simulink model "SPath"  (R2020a)
settings: Solver=VariableStepAuto  StartTime=0.0  StopTime=150  RelTol=1e-3
values from neighbouring files (symbols this model uses):
  b = 0.4    [Takeoff.m]
  body_rate_0 = [0;0;0]    [Takeoff.m]
  Boundaries = [B1;B2;B3]    [Takeoff.m]
  Euler_0 = [0;0;0]    [Takeoff.m]
  g = [0;0;-9.8]    [Takeoff.m]
  I_Drone = [0.3933,0.3933,0.76]    [Takeoff.m]
  I_Tank = CalItank(m_tank,0.4,0.1,0.4,i)    [Takeoff.m]
  J = 0.00062    [Takeoff.m]
  K = 0.074    [Takeoff.m]
  k_T = MaxMotorThrsut/(MaxRPM^2)    (= 6.99167657551e-06)    [Takeoff.m]
  k_Thrsut2Torque = 0.021    [Takeoff.m]
  l = 0.5    [Takeoff.m]
  L = sqrt((x2-x1)^2 + (y2-y1)^2)    [Takeoff.m]
  m = m_drone + m_tank*percent    (= 36)    [Takeoff.m]    (also in animation.m = T_V1toI*T_V2toV1*T_BtoV2)
  m_drone = 20    [Takeoff.m]
  m_tank = 16    [Takeoff.m]
  MaxThrust = 4*MaxMotorThrsut    (= 529.2)    [Takeoff.m]
  MaxTilt = 30*pi/180    (= 0.523598775598)    [Takeoff.m]
  MaxTorque_XY = (T2-T1)*(l/sqrt(2))    [Takeoff.m]
  MaxVolt = 48    [Takeoff.m]
  MaxYawRate = 100*pi/180    (= 1.74532925199)    [Takeoff.m]
  MaxZVel = 2    [Takeoff.m]
  percent = 1    [Takeoff.m]
  Px1 = 0.2    [Takeoff.m]
  Pz1 = 1    [Takeoff.m]
  Pz2 = 100    [Takeoff.m]
  R = 0.0062    [Takeoff.m]
  SafeZone = 1.0    (= 1)    [Takeoff.m]
  ts = 0.01    [Takeoff.m]
  WayPts = [[XYZ_0(1) XYZ_0(2) XYZ_0(3)] ... (first row only)    [Takeoff.m]
  XYZ_0 = [0;0;0]    [Takeoff.m]
undefined symbols (not defined in the file or in its folder): b_tank, d_drone, d_tank, DiscIntNeverNeededParam, FlyVel, h_tank, NWay, PD1, PD2, PI1, PI2, PP1, PP2, Sensor0Dir, ts_out, WayPtsYaw
libraries: simulink x26, vrlib x4, simulink_extras x2
(part 3 of 3)

== system SPath/Controller/Rotors System1/Propellers/Motor Thrust Control2 ==
  Ref_Thrust : Inport
  DC Motor : Subsystem
  Gain2 : Gain  Gain=k_T
  Gain3 : Gain  Gain=1/k_T
  Gain4 : Gain  Gain=30/pi
  MATLAB Function : MATLAB Function  TreatAsAtomicUnit=on
  PID Controller : simulink/Continuous/PID Controller  Controller=PI  Form=Parallel  TimeDomain=Discrete-time  UseExternalTs=off  SampleTime=ts  IntegratorMethod=Forward Euler  FilterMethod=Forward Euler  ControllerParametersSource=internal  P=0.005  I=0.5  D=0.01  UseFilter=on  N=100  TunerSelectOption=Transfer Function Based (PID Tuner App)  InitialConditionSource=internal  InitialConditionForIntegrator=0  InitialConditionForFilter=0  DifferentiatorICPrevScaledInput=0  ExternalReset=none  TrackingMode=off  Kt=1  LimitOutput=off  UpperSaturationLimit=inf  LowerSaturationLimit=-inf  LinearizeAsGain=on  AntiWindupMode=none  Kb=1  POutMin=[]  POutMax=[]  IOutMin=[]  IOutMax=[]  DOutMin=[]  DOutMax=[]  NOutMin=[]  NOutMax=[]  SumOutMin=[]  SumOutMax=[]  SaturationOutMin=[]  SaturationOutMax=[]  PParamMin=[]  PParamMax=[]  IParamMin=[]  IParamMax=[]  DParamMin=[]  DParamMax=[]  NParamMin=[]  NParamMax=[]  KbParamMin=[]  KbParamMax=[]  KtParamMin=[]  KtParamMax=[]  KbOutMin=[]  KbOutMax=[]  KtOutMin=[]  KtOutMax=[]  IntegratorOutMin=[]  IntegratorOutMax=[]  FilterOutMin=[]  FilterOutMax=[]  SumI1OutMin=[]  SumI1OutMax=[]  SumI2OutMin=[]  SumI2OutMax=[]  SumI3OutMin=[]  SumI3OutMax=[]  SumI4OutMin=[]  SumI4OutMax=[]  SumDOutMin=[]  SumDOutMax=[]  DifferentiatorOutMin=[]  DifferentiatorOutMax=[]  FilterDiffOutCoefMin=[]  FilterDiffOutCoefMax=[]  ReciprocalOutMin=[]  ReciprocalOutMax=[]  SumDenOutMin=[]  SumDenOutMax=[]  SumNumOutMin=[]  SumNumOutMax=[]  DivideOutMin=[]  DivideOutMax=[]  UdiffTsProdOutMin=[]  UdiffTsProdOutMax=[]  NTsProdOutMin=[]  NTsProdOutMax=[]  UintegralTsProdOutMin=[]  UintegralTsProdOutMax=[]  UngainTsProdOutMin=[]  UngainTsProdOutMax=[]  IntegratorContinuousStateAttributes=''  IntegratorStateMustResolveToSignalObject=off  IntegratorRTWStateStorageClass=Auto  FilterContinuousStateAttributes=''  FilterStateMustResolveToSignalObject=off  FilterRTWStateStorageClass=Auto  ParallelPVariant=InternalParameters  IdealPVariant=Disabled  IVariant=InternalParameters  DVariant=Disabled  IntegratorVariant=Discrete  SatVariant=Disabled  AWVariant=Passthrough  PCopyVariant=Disabled  TRVariant=Disabled  FdbkBlocksVariant=Forward  IdealPFdbkVariant=Disabled  SatFdbkVariant=Disabled  DerivativeFilterVariant=Disabled  NVariant=Disabled  NCopyVariant=Disabled_SignalSpec  FilterICVariant=Disabled  IntegratorICVariant=InternalICs  ExternalResetVariant=Disabled  TRSumVariant=Passthrough  SumFdbkVariant=Disabled  SumVariant=Sum_PI  TsampFilterVariant=InternalTs  TsampNgainVariant=Passthrough  TsampIntegralVariant=Passthrough
  PID Controller1 : simulink/Continuous/PID Controller  Commented=on  Controller=PID  Form=Parallel  TimeDomain=Discrete-time  UseExternalTs=off  SampleTime=ts  IntegratorMethod=Forward Euler  FilterMethod=Forward Euler  ControllerParametersSource=internal  P=69.4635476284255  I=231.449566152495  D=-0.149403920537339  UseFilter=on  N=139.13500041138  TunerSelectOption=Transfer Function Based (PID Tuner App)  InitialConditionSource=internal  InitialConditionForIntegrator=0  InitialConditionForFilter=0  DifferentiatorICPrevScaledInput=0  ExternalReset=none  TrackingMode=off  Kt=1  LimitOutput=off  UpperSaturationLimit=inf  LowerSaturationLimit=-inf  LinearizeAsGain=on  AntiWindupMode=none  Kb=1  POutMin=[]  POutMax=[]  IOutMin=[]  IOutMax=[]  DOutMin=[]  DOutMax=[]  NOutMin=[]  NOutMax=[]  SumOutMin=[]  SumOutMax=[]  SaturationOutMin=[]  SaturationOutMax=[]  PParamMin=[]  PParamMax=[]  IParamMin=[]  IParamMax=[]  DParamMin=[]  DParamMax=[]  NParamMin=[]  NParamMax=[]  KbParamMin=[]  KbParamMax=[]  KtParamMin=[]  KtParamMax=[]  KbOutMin=[]  KbOutMax=[]  KtOutMin=[]  KtOutMax=[]  IntegratorOutMin=[]  IntegratorOutMax=[]  FilterOutMin=[]  FilterOutMax=[]  SumI1OutMin=[]  SumI1OutMax=[]  SumI2OutMin=[]  SumI2OutMax=[]  SumI3OutMin=[]  SumI3OutMax=[]  SumI4OutMin=[]  SumI4OutMax=[]  SumDOutMin=[]  SumDOutMax=[]  DifferentiatorOutMin=[]  DifferentiatorOutMax=[]  FilterDiffOutCoefMin=[]  FilterDiffOutCoefMax=[]  ReciprocalOutMin=[]  ReciprocalOutMax=[]  SumDenOutMin=[]  SumDenOutMax=[]  SumNumOutMin=[]  SumNumOutMax=[]  DivideOutMin=[]  DivideOutMax=[]  UdiffTsProdOutMin=[]  UdiffTsProdOutMax=[]  NTsProdOutMin=[]  NTsProdOutMax=[]  UintegralTsProdOutMin=[]  UintegralTsProdOutMax=[]  UngainTsProdOutMin=[]  UngainTsProdOutMax=[]  IntegratorContinuousStateAttributes=''  IntegratorStateMustResolveToSignalObject=off  IntegratorRTWStateStorageClass=Auto  FilterContinuousStateAttributes=''  FilterStateMustResolveToSignalObject=off  FilterRTWStateStorageClass=Auto  ParallelPVariant=InternalParameters  IdealPVariant=Disabled  IVariant=InternalParameters  DVariant=InternalParameters  IntegratorVariant=Discrete  SatVariant=Disabled  AWVariant=Passthrough  PCopyVariant=Disabled  TRVariant=Disabled  FdbkBlocksVariant=Forward  IdealPFdbkVariant=Disabled  SatFdbkVariant=Disabled  DerivativeFilterVariant=ForwardEulerFilter  NVariant=InternalParameters  NCopyVariant=Disabled  FilterICVariant=InternalICsFilter  IntegratorICVariant=InternalICs  ExternalResetVariant=Disabled  TRSumVariant=Passthrough  SumFdbkVariant=Disabled  SumVariant=Sum_PID  TsampFilterVariant=InternalTs  TsampNgainVariant=Passthrough  TsampIntegralVariant=Passthrough
  Rate Transition : RateTransition  OutPortSampleTime=ts
  Saturation1 : Saturate  Commented=on  UpperLimit=MaxVolt  LowerLimit=-MaxVolt
  Scope : Scope
  Scope1 : Scope
  Square : Math  Operator=square  SaturateOnIntegerOverflow=on
  Square Root : Sqrt  SaturateOnIntegerOverflow=on
  Sum : Sum  Inputs=|+-
  Transfer Fcn1 : TransferFcn  Commented=on  Numerator=[44 44]  Denominator=[1 0.01]
  Thrust : Outport
  wires:
  MATLAB Function/1(y) -> DC Motor/2(TQ_load)
  Sum/1 -> PID Controller/1
  Square Root/1 -> Sum/1  "Ref_RPM"
  PID Controller/1 -> DC Motor/1(Voltage)
  Gain4/1 -> Scope/1, Square/1, Rate Transition/1, MATLAB Function/1(u)  "RPM"
  DC Motor/1(Speed) -> Gain4/1
  Rate Transition/1 -> Sum/2
  Gain2/1 -> Thrust/1, Scope1/1  "Thrust"
  Ref_Thrust/1 -> Gain3/1
  Square/1 -> Gain2/1
  Gain3/1 -> Square Root/1

== system SPath/Controller/Rotors System1/Propellers/Motor Thrust Control3 ==
  Ref_Thrust : Inport
  DC Motor : Subsystem
  Gain2 : Gain  Gain=k_T
  Gain3 : Gain  Gain=1/k_T
  Gain4 : Gain  Gain=30/pi
  MATLAB Function : MATLAB Function  TreatAsAtomicUnit=on
  PID Controller : simulink/Continuous/PID Controller  Controller=PI  Form=Parallel  TimeDomain=Discrete-time  UseExternalTs=off  SampleTime=ts  IntegratorMethod=Forward Euler  FilterMethod=Forward Euler  ControllerParametersSource=internal  P=0.005  I=0.5  D=0.01  UseFilter=on  N=100  TunerSelectOption=Transfer Function Based (PID Tuner App)  InitialConditionSource=internal  InitialConditionForIntegrator=0  InitialConditionForFilter=0  DifferentiatorICPrevScaledInput=0  ExternalReset=none  TrackingMode=off  Kt=1  LimitOutput=off  UpperSaturationLimit=inf  LowerSaturationLimit=-inf  LinearizeAsGain=on  AntiWindupMode=none  Kb=1  POutMin=[]  POutMax=[]  IOutMin=[]  IOutMax=[]  DOutMin=[]  DOutMax=[]  NOutMin=[]  NOutMax=[]  SumOutMin=[]  SumOutMax=[]  SaturationOutMin=[]  SaturationOutMax=[]  PParamMin=[]  PParamMax=[]  IParamMin=[]  IParamMax=[]  DParamMin=[]  DParamMax=[]  NParamMin=[]  NParamMax=[]  KbParamMin=[]  KbParamMax=[]  KtParamMin=[]  KtParamMax=[]  KbOutMin=[]  KbOutMax=[]  KtOutMin=[]  KtOutMax=[]  IntegratorOutMin=[]  IntegratorOutMax=[]  FilterOutMin=[]  FilterOutMax=[]  SumI1OutMin=[]  SumI1OutMax=[]  SumI2OutMin=[]  SumI2OutMax=[]  SumI3OutMin=[]  SumI3OutMax=[]  SumI4OutMin=[]  SumI4OutMax=[]  SumDOutMin=[]  SumDOutMax=[]  DifferentiatorOutMin=[]  DifferentiatorOutMax=[]  FilterDiffOutCoefMin=[]  FilterDiffOutCoefMax=[]  ReciprocalOutMin=[]  ReciprocalOutMax=[]  SumDenOutMin=[]  SumDenOutMax=[]  SumNumOutMin=[]  SumNumOutMax=[]  DivideOutMin=[]  DivideOutMax=[]  UdiffTsProdOutMin=[]  UdiffTsProdOutMax=[]  NTsProdOutMin=[]  NTsProdOutMax=[]  UintegralTsProdOutMin=[]  UintegralTsProdOutMax=[]  UngainTsProdOutMin=[]  UngainTsProdOutMax=[]  IntegratorContinuousStateAttributes=''  IntegratorStateMustResolveToSignalObject=off  IntegratorRTWStateStorageClass=Auto  FilterContinuousStateAttributes=''  FilterStateMustResolveToSignalObject=off  FilterRTWStateStorageClass=Auto  ParallelPVariant=InternalParameters  IdealPVariant=Disabled  IVariant=InternalParameters  DVariant=Disabled  IntegratorVariant=Discrete  SatVariant=Disabled  AWVariant=Passthrough  PCopyVariant=Disabled  TRVariant=Disabled  FdbkBlocksVariant=Forward  IdealPFdbkVariant=Disabled  SatFdbkVariant=Disabled  DerivativeFilterVariant=Disabled  NVariant=Disabled  NCopyVariant=Disabled_SignalSpec  FilterICVariant=Disabled  IntegratorICVariant=InternalICs  ExternalResetVariant=Disabled  TRSumVariant=Passthrough  SumFdbkVariant=Disabled  SumVariant=Sum_PI  TsampFilterVariant=InternalTs  TsampNgainVariant=Passthrough  TsampIntegralVariant=Passthrough
  PID Controller1 : simulink/Continuous/PID Controller  Commented=on  Controller=PID  Form=Parallel  TimeDomain=Discrete-time  UseExternalTs=off  SampleTime=ts  IntegratorMethod=Forward Euler  FilterMethod=Forward Euler  ControllerParametersSource=internal  P=69.4635476284255  I=231.449566152495  D=-0.149403920537339  UseFilter=on  N=139.13500041138  TunerSelectOption=Transfer Function Based (PID Tuner App)  InitialConditionSource=internal  InitialConditionForIntegrator=0  InitialConditionForFilter=0  DifferentiatorICPrevScaledInput=0  ExternalReset=none  TrackingMode=off  Kt=1  LimitOutput=off  UpperSaturationLimit=inf  LowerSaturationLimit=-inf  LinearizeAsGain=on  AntiWindupMode=none  Kb=1  POutMin=[]  POutMax=[]  IOutMin=[]  IOutMax=[]  DOutMin=[]  DOutMax=[]  NOutMin=[]  NOutMax=[]  SumOutMin=[]  SumOutMax=[]  SaturationOutMin=[]  SaturationOutMax=[]  PParamMin=[]  PParamMax=[]  IParamMin=[]  IParamMax=[]  DParamMin=[]  DParamMax=[]  NParamMin=[]  NParamMax=[]  KbParamMin=[]  KbParamMax=[]  KtParamMin=[]  KtParamMax=[]  KbOutMin=[]  KbOutMax=[]  KtOutMin=[]  KtOutMax=[]  IntegratorOutMin=[]  IntegratorOutMax=[]  FilterOutMin=[]  FilterOutMax=[]  SumI1OutMin=[]  SumI1OutMax=[]  SumI2OutMin=[]  SumI2OutMax=[]  SumI3OutMin=[]  SumI3OutMax=[]  SumI4OutMin=[]  SumI4OutMax=[]  SumDOutMin=[]  SumDOutMax=[]  DifferentiatorOutMin=[]  DifferentiatorOutMax=[]  FilterDiffOutCoefMin=[]  FilterDiffOutCoefMax=[]  ReciprocalOutMin=[]  ReciprocalOutMax=[]  SumDenOutMin=[]  SumDenOutMax=[]  SumNumOutMin=[]  SumNumOutMax=[]  DivideOutMin=[]  DivideOutMax=[]  UdiffTsProdOutMin=[]  UdiffTsProdOutMax=[]  NTsProdOutMin=[]  NTsProdOutMax=[]  UintegralTsProdOutMin=[]  UintegralTsProdOutMax=[]  UngainTsProdOutMin=[]  UngainTsProdOutMax=[]  IntegratorContinuousStateAttributes=''  IntegratorStateMustResolveToSignalObject=off  IntegratorRTWStateStorageClass=Auto  FilterContinuousStateAttributes=''  FilterStateMustResolveToSignalObject=off  FilterRTWStateStorageClass=Auto  ParallelPVariant=InternalParameters  IdealPVariant=Disabled  IVariant=InternalParameters  DVariant=InternalParameters  IntegratorVariant=Discrete  SatVariant=Disabled  AWVariant=Passthrough  PCopyVariant=Disabled  TRVariant=Disabled  FdbkBlocksVariant=Forward  IdealPFdbkVariant=Disabled  SatFdbkVariant=Disabled  DerivativeFilterVariant=ForwardEulerFilter  NVariant=InternalParameters  NCopyVariant=Disabled  FilterICVariant=InternalICsFilter  IntegratorICVariant=InternalICs  ExternalResetVariant=Disabled  TRSumVariant=Passthrough  SumFdbkVariant=Disabled  SumVariant=Sum_PID  TsampFilterVariant=InternalTs  TsampNgainVariant=Passthrough  TsampIntegralVariant=Passthrough
  Rate Transition : RateTransition  OutPortSampleTime=ts
  Saturation1 : Saturate  Commented=on  UpperLimit=MaxVolt  LowerLimit=-MaxVolt
  Scope : Scope
  Scope1 : Scope
  Square : Math  Operator=square  SaturateOnIntegerOverflow=on
  Square Root : Sqrt  SaturateOnIntegerOverflow=on
  Sum : Sum  Inputs=|+-
  Transfer Fcn1 : TransferFcn  Commented=on  Numerator=[44 44]  Denominator=[1 0.01]
  Thrust : Outport
  wires:
  Gain3/1 -> Square Root/1
  Square/1 -> Gain2/1
  Ref_Thrust/1 -> Gain3/1
  Gain2/1 -> Scope1/1, Thrust/1  "Thrust"
  Rate Transition/1 -> Sum/2
  DC Motor/1(Speed) -> Gain4/1
  Gain4/1 -> MATLAB Function/1(u), Rate Transition/1, Square/1, Scope/1  "RPM"
  PID Controller/1 -> DC Motor/1(Voltage)
  Square Root/1 -> Sum/1  "Ref_RPM"
  Sum/1 -> PID Controller/1
  MATLAB Function/1(y) -> DC Motor/2(TQ_load)

== system SPath/Controller/Rotors System1/Propellers/Motor Thrust Control/Brushless DC Motor ==
  note: d2/dt2(theta)
  note: d/dt(theta)
  note: d/dt(i)
  note: i
  Voltage : Inport
  TQ_load : Inport  Port=2
  Add : Sum  Inputs=-+-
  Add1 : Sum  Inputs=+--
  Damping : Gain  Gain=b
  Inductance : Gain  Gain=1/L
  Inertia : Gain  Gain=1/J
  Integrator : Integrator
  Integrator1 : Integrator
  Ke : Gain  Gain=K
  Kt : Gain  Gain=K
  Resistance : Gain  Gain=R
  Scope : Scope  NumInputPorts=2
  Speed : Outport
  wires:
  TQ_load/1 -> Add1/3
  Add1/1 -> Inertia/1
  Add/1 -> Inductance/1
  Ke/1 -> Add/3
  Damping/1 -> Add1/2
  Resistance/1 -> Add/1
  Voltage/1 -> Add/2
  Kt/1 -> Add1/1
  Integrator/1 -> Resistance/1, Scope/1, Kt/1
  Inertia/1 -> Integrator1/1
  Integrator1/1 -> Ke/1, Speed/1, Scope/2, Damping/1
  Inductance/1 -> Integrator/1

== system SPath/Controller/Rotors System1/Propellers/Motor Thrust Control1/DC Motor ==
  note: i
  note: d/dt(i)
  note: d/dt(theta)
  note: d2/dt2(theta)
  Voltage : Inport
  TQ_load : Inport  Port=2
  Add : Sum  Inputs=-+-
  Add1 : Sum  Inputs=+--
  Damping : Gain  Gain=b
  Inductance : Gain  Gain=1/L
  Inertia : Gain  Gain=1/J
  Integrator : Integrator
  Integrator1 : Integrator
  Ke : Gain  Gain=K
  Kt : Gain  Gain=K
  Resistance : Gain  Gain=R
  Scope : Scope  NumInputPorts=2
  Speed : Outport
  wires:
  Inductance/1 -> Integrator/1
  Integrator1/1 -> Damping/1, Scope/2, Speed/1, Ke/1
  Inertia/1 -> Integrator1/1
  Integrator/1 -> Kt/1, Scope/1, Resistance/1
  Kt/1 -> Add1/1
  Voltage/1 -> Add/2
  Resistance/1 -> Add/1
  Damping/1 -> Add1/2
  Ke/1 -> Add/3
  Add/1 -> Inductance/1
  Add1/1 -> Inertia/1
  TQ_load/1 -> Add1/3

== system SPath/Controller/Rotors System1/Propellers/Motor Thrust Control2/DC Motor ==
  note: d2/dt2(theta)
  note: d/dt(theta)
  note: d/dt(i)
  note: i
  Voltage : Inport
  TQ_load : Inport  Port=2
  Add : Sum  Inputs=-+-
  Add1 : Sum  Inputs=+--
  Damping : Gain  Gain=b
  Inductance : Gain  Gain=1/L
  Inertia : Gain  Gain=1/J
  Integrator : Integrator
  Integrator1 : Integrator
  Ke : Gain  Gain=K
  Kt : Gain  Gain=K
  Resistance : Gain  Gain=R
  Scope : Scope  NumInputPorts=2
  Speed : Outport
  wires:
  TQ_load/1 -> Add1/3
  Add1/1 -> Inertia/1
  Add/1 -> Inductance/1
  Ke/1 -> Add/3
  Damping/1 -> Add1/2
  Resistance/1 -> Add/1
  Voltage/1 -> Add/2
  Kt/1 -> Add1/1
  Integrator/1 -> Resistance/1, Scope/1, Kt/1
  Inertia/1 -> Integrator1/1
  Integrator1/1 -> Ke/1, Speed/1, Scope/2, Damping/1
  Inductance/1 -> Integrator/1

== system SPath/Controller/Rotors System1/Propellers/Motor Thrust Control3/DC Motor ==
  note: i
  note: d/dt(i)
  note: d/dt(theta)
  note: d2/dt2(theta)
  Voltage : Inport
  TQ_load : Inport  Port=2
  Add : Sum  Inputs=-+-
  Add1 : Sum  Inputs=+--
  Damping : Gain  Gain=b
  Inductance : Gain  Gain=1/L
  Inertia : Gain  Gain=1/J
  Integrator : Integrator
  Integrator1 : Integrator
  Ke : Gain  Gain=K
  Kt : Gain  Gain=K
  Resistance : Gain  Gain=R
  Scope : Scope  NumInputPorts=2
  Speed : Outport
  wires:
  Inductance/1 -> Integrator/1
  Integrator1/1 -> Damping/1, Scope/2, Speed/1, Ke/1
  Inertia/1 -> Integrator1/1
  Integrator/1 -> Kt/1, Scope/1, Resistance/1
  Kt/1 -> Add1/1
  Voltage/1 -> Add/2
  Resistance/1 -> Add/1
  Damping/1 -> Add1/2
  Ke/1 -> Add/3
  Add/1 -> Inductance/1
  Add1/1 -> Inertia/1
  TQ_load/1 -> Add1/3

== matlab function SPath/Controller/Rotors System1/Propellers/Motor Thrust Control/MATLAB Function ==
  data: u input; y output
function y = fcn(u)
    y = 0.000009*u^2;

    % The coefficient is decided by experimental value.
    % Max RPM = 4350, 48 Volt.

== matlab function SPath/Controller/Rotors System1/Propellers/Motor Thrust Control1/MATLAB Function ==
  data: u input; y output
function y = fcn(u)
    y = 0.000009*u^2;

    % The coefficient is decided by experimental value.
    % Max RPM = 4350, 48 Volt.

== matlab function SPath/Controller/Rotors System1/Propellers/Motor Thrust Control2/MATLAB Function ==
  data: u input; y output
function y = fcn(u)
    y = 0.000009*u^2;

    % The coefficient is decided by experimental value.
    % Max RPM = 4350, 48 Volt.

== matlab function SPath/6dof_system/Drone & Liquid Dynamic Inertia/DroneTankI ==
  data: I_D input; I output; I_T input; M_D input; M_T input; Z_D input; Z_T input; CR_X input; CR_Y input
function I = fcn(I_D,I_T,M_D,M_T,Z_D,Z_T,CR_X,CR_Y)

    Ix = I_D(1) + M_D*Z_D^2 + CR_X*I_T(1) + M_T*Z_T^2;
    Iy = I_D(2) + M_D*Z_D^2 + CR_Y*I_T(2) + M_T*Z_T^2;
    Iz = I_D(3) + I_T(3);
    I = [[Ix 0 0];[0 Iy 0];[0 0 Iz]];

== matlab function SPath/6dof_system/Drone & Liquid Dynamic Inertia/FullTankCR ==
  data: w_d input; CR_x output; CR_y output; C_R input
function [CR_x,CR_y] = fcn(w_d,C_R)
if length(w_d) > 1
    if abs(w_d(2)) > 0.001
        CR_y = C_R;
    else
        CR_y = 1;
    end
    
    if abs(w_d(1)) > 0.001
        CR_x = C_R;
    else
        CR_x = 1;
    end
else
    CR_x = 1;
    CR_y = 1;
end

== matlab function SPath/Controller/Rotors System1/Propellers/Motor Thrust Control3/MATLAB Function ==
  data: u input; y output
function y = fcn(u)
    y = 0.000009*u^2;

    % The coefficient is decided by experimental value.
    % Max RPM = 4350, 48 Volt.

== matlab function SPath/Controller/ActionDecider/SlowDown_Detect/SlowDown_Detect ==
  data: mode input; D_SD input; D_SF input; S0X input; action output; S0Y input; S1X input; S2X input
function action = fcn(mode,D_SD,D_SF,S0X,S0Y,S1X,S2X)
action = 0;
if mode == 0     
    
    if abs(S0X) <= D_SD && abs(S0Y) <= 1.5*D_SF
        action = 1;
    end
    
end

== matlab function SPath/Controller/Sensors/Sensor0 (15 degree sensor) ==
  data: Pos input; MinBDist output; Bounds input; Yaw input; MinBVect output; Directions input; RightVect output; MinRight output; LeftVect output; MinLeft output
function [MinBDist,MinBVect,RightVect,MinRight,LeftVect,MinLeft] = fcn(Pos,Bounds,Yaw,Directions)
MaxRange = 30;
MinBDist = MaxRange;
m = [[cos(Yaw) -sin(Yaw)];[sin(Yaw) cos(Yaw)]];
nn = m*[1;0];
MinBVect = [nn(1);nn(2);0];

% For Visual
RightVect = MinBVect;
MinRight = MaxRange;
LeftVect = MinBVect;
MinLeft = MaxRange;

RightDist = MaxRange;
LeftDist = MaxRange;

for b = 1:size(Bounds,1)
Bound = Bounds(b,:);

%Bound = Bounds(BIndex,:);
MinSenseDist = MaxRange;
m = [[cos(Yaw) -sin(Yaw)];[sin(Yaw) cos(Yaw)]];
nnn = m*[1;0];
MinSenseVect = [nnn(1);nnn(2);0];




for k = 1:size(Directions,2)
if length(Pos) > 1
    bx = Bound(1);
    by = Bound(2);
    tx = Bound(3);
    ty = Bound(4);
    X = Pos(1);
    Y = Pos(2);
    Z = Pos(3);
    
    m = [[cos(Yaw) -sin(Yaw)];[sin(Yaw) cos(Yaw)]];
    nn = m*Directions(:,k); % Sense vector in Inertia Frame
    nx = nn(1);
    ny = nn(2);

    j = ((ty*bx-tx*by)-(ty*X-tx*Y))/(ty*nx-tx*ny);
    
    if j < 0 % sense backward point
        SenseDist = MaxRange;
    else
        SensePt = [X+nx*j;Y+ny*j];
        
        % Check if ON boundaries
        if tx == 0
            i = (SensePt(2)-by)/ty;
        else
            i = (SensePt(1)-bx)/tx;
        end
        
        % If not
        if i < 0 || i > Bound(7)
            SenseDist = MaxRange;
        % If yes
        else
            SenseDist = sqrt((nx*j)^2 + (ny*j)^2);
        end
    end
    
    % Calculate Directions
    SenseVect = [nx;ny;0]/sqrt(nx^2+ny^2);
    
else
    SenseDist = MaxRange;
    SenseVect = [0;0;0];
end

if SenseDist < MinSenseDist
    MinSenseDist = SenseDist;
    MinSenseVect = SenseVect;
end

% Collect Right and Left Bounds Vector for Visual
if k == 1
    RightVect = SenseVect;
    RightDist = SenseDist;
end
if k == size(Directions,2)
    LeftVect = SenseVect;
    LeftDist = SenseDist;
end


end % end of -15:1:15 for loop


if MinSenseDist < MinBDist
    MinBDist = MinSenseDist;
    MinBVect = MinSenseVect;
end


if RightDist < MinRight
    MinRight = RightDist;
end

if LeftDist < MinLeft
    MinLeft = LeftDist;
end


end

== matlab function SPath/Controller/FlyModeCmd/SlowDown Fly ==
  data: mode input; XVelCmd output; V_AO input
function XVelCmd = fcn(mode,V_AO)
% Mode 1: SlowDown Fly
XVelCmd = 0;
if mode == 1
    XVelCmd = V_AO;
end

== matlab function SPath/Controller/FlyModeCmd/FM Fly ==
  data: mode input; YVelCmd output; V_AO input; FM_Dir input
function YVelCmd = fcn(mode,V_AO,FM_Dir)
% Mode 2: First Maneuver Fly
YVelCmd = 0;
if mode == 2
    YVelCmd = FM_Dir*V_AO;
end

== matlab function SPath/Controller/Sensors/MATLAB Function ==
  data: Vect input; Vect_Body output; Yaw input
function Vect_Body = fcn(Vect,Yaw)
if length(Vect) > 1
    m = [[cos(Yaw) -sin(Yaw) 0];[sin(Yaw) cos(Yaw) 0]; [0 0 1]];
    m = transpose(m);
    Vect_Body = m*[Vect(1);Vect(2);0];
else
    Vect_Body = [1;0;0];
end

== matlab function SPath/Controller/ActionDecider/FirstManeuver_Detect/FM_Detect ==
  data: mode input; S0X input; S0Y input; action output; S1X input; S2X input; FM_Dir output; HotFix output; timeM1 input
function [action,FM_Dir,HotFix] = fcn(mode,S0X,S0Y,S1X,S2X,timeM1)
action = 0;
FM_Dir = 0;

MaxRange = 5;

%HotFix
HotFix = 0;

if mode == 1     
    if S0X <= 2.2 && timeM1 > 0.5 %2.5*D_SF + D_DR
        action = 1;
        
        % Decide Direction
        if S1X ~= MaxRange && S2X ~= MaxRange
            if S0Y < 0 % Something at Right
                FM_Dir = 1;    % Left Body Dir (1)
                HotFix = 1;
            else
                FM_Dir = -1;   % Right Body Dir
                HotFix = 1;
            end
            return;        
        end
        
        if S1X == MaxRange || S2X == MaxRange
            if S1X < MaxRange
                FM_Dir = 1; %(1 for left)
                HotFix = 1;
                
            elseif S2X < MaxRange
                FM_Dir = -1;
                HotFix = 1;
                
            else
                if S0Y < 0 % Something at Right
                    FM_Dir = 1;    % Left Body Dir (1)
                    
                    % Hot Fix for Extreme Case.
                    if abs(S0Y) >=  0.5*cos(45*pi/180)
                        HotFix = 1;
                    end
                else
                    FM_Dir = -1;   % Right Body Dir
                    
                    % Hot Fix for Extreme Case.
                    if abs(S0Y) >=  0.5*cos(45*pi/180)
                        HotFix = 1;
                    end
                end
            end
        end
        
    end  
    
    
    % Robust Algo: SlowDown but don't avoid: go to Normal Fly
    if S0X >= 20
        action = -1;
    end
    
end

== matlab function SPath/Controller/ActionDecider/SecondManeuver_Detect/XTouch_Detect ==
  data: mode input; Flag output; S1X input; S2X input; D_SF input; FM_Dir input
function Flag = fcn(mode,S1X,S2X,D_SF,FM_Dir)
Flag = 0;
if mode == 2
    if FM_Dir == -1 && S2X < 3*D_SF
        Flag = 1;
        return;
    end
    
    if FM_Dir == 1 && S1X < 3*D_SF
        Flag = 1;
        return;
    end
end

== matlab function SPath/6dof_system/BtoITransform ==
  data: phi input; m output; theta input; psi input
function m = fcn(phi,theta,psi)
    T_BtoV2 = [[1 0 0];[0 cos(-phi) sin(-phi)];[0 -sin(-phi) cos(-phi)]];
    T_V2toV1 = [[cos(-theta) 0 -sin(-theta)];[0 1 0];[sin(-theta) 0 cos(-theta)]];
    T_V1toI = [[cos(-psi) sin(-psi) 0];[-sin(-psi) cos(-psi) 0];[0 0 1]];
    m = T_V1toI*T_V2toV1*T_BtoV2;

== matlab function SPath/Controller/ActionDecider/SecondManeuver_Detect/SM_Detect ==
  data: mode input; timer1 input; action output; t_bf1 input
function action = fcn(mode,timer1,t_bf1)
action = 0;
if mode == 2 && timer1 >= t_bf1
    action = 1;
end

== matlab function SPath/Select WayPoint/ChooseTarget ==
  data: WayPts input; WayPtsYaw input; TargetWayPts output; WayPtsIndex input; TargetWayPtsYaw output; number input
function [TargetWayPts,TargetWayPtsYaw] = fcn(WayPts,WayPtsYaw,WayPtsIndex,number)
if WayPtsIndex < number
    TargetWayPts = WayPts(WayPtsIndex+1,:);
    TargetWayPtsYaw = WayPtsYaw(WayPtsIndex+1);
else
    TargetWayPts = WayPts(number,:);
    TargetWayPtsYaw = WayPtsYaw(number);
end

== matlab function SPath/Select WayPoint/IsReachTarget ==
  data: XYZe input; TouchWayPts output; Yawe input; Index input; time input; number input; Speed input
function TouchWayPts = fcn(XYZe,Yawe,Index,time,number,Speed)
TouchWayPts = 0;

if Index == 0
    if XYZe < 0.1
        TouchWayPts = 1;
    end
elseif Index == 1
    if time >= 5
        TouchWayPts = 1;
    end
elseif Index >= number
    TouchWayPts = 0;
else
    if XYZe < 0.1 && Yawe < 0.05 %&& Speed < 0.5
        TouchWayPts = 1;
    end  
end

== matlab function SPath/Controller/ActionDecider/SecondManeuver_Detect/Crossover_Detect ==
  data: mode input; IsTouchX input; S1X input; count output; S2X input; FM_Dir input; D_SF input
function count = fcn(mode,IsTouchX,S1X,S2X,FM_Dir,D_SF)
count = 0;

% HotFix
MaxRange = 5;

if mode == 2
if FM_Dir == -1
    if IsTouchX == 1 && S2X >= MaxRange
        count = 1;
        return;
    end
end

if FM_Dir == 1
    if IsTouchX == 1 && S1X >= MaxRange
        count = 1;
        return;
    end
end
end

== matlab function SPath/Controller/FlyModeCmd/SM Fly ==
  data: mode input; XVelCmd output; V_AO input
function XVelCmd = fcn(mode,V_AO)
% Mode 3: Second Maneuver Fly
XVelCmd = 0;
if mode == 3
    XVelCmd = V_AO;
end

== matlab function SPath/Controller/ActionDecider/Recover_Detect/Crossover_Detect ==
  data: mode input; IsTouchY input; S1Y input; count output; S2Y input; FM_Dir input; D_SF input
function count = fcn(mode,IsTouchY,S1Y,S2Y,FM_Dir,D_SF)
count = 0;
if mode == 3
if FM_Dir == -1
    if IsTouchY == 1 && S2Y > 2*D_SF
        count = 1;
        return;
    end
end

if FM_Dir == 1
    if IsTouchY == 1 && S1Y > 2*D_SF
        count = 1;
        return;
    end
end
end

== matlab function SPath/Controller/ActionDecider/Recover_Detect/TM_Detect ==
  data: mode input; timer2 input; action output; t_bf2 input
function action = fcn(mode,timer2,t_bf2)
action = 0;
if mode == 3 && timer2 >= t_bf2
    action = 1;
end

== matlab function SPath/Controller/ActionDecider/Recover_Detect/YTouch_Detect ==
  data: mode input; Flag output; S1Y input; S2Y input; D_SF input; FM_Dir input
function Flag = fcn(mode,S1Y,S2Y,D_SF,FM_Dir)
Flag = 0;
if mode == 3
    if FM_Dir == -1 && S2Y < 3*D_SF
        Flag = 1;
        return;
    end
    
    if FM_Dir == 1 && S1Y < 3*D_SF
        Flag = 1;
        return;
    end
end

== matlab function SPath/Controller/FlyModeCmd/Recover Fly ==
  data: mode input; YVelCmd output; V_AO input; FM_Dir input
function YVelCmd = fcn(mode,V_AO,FM_Dir)
% Mode 4: Recover Fly
YVelCmd = 0;
if mode == 4
    YVelCmd = -FM_Dir*V_AO;
end

== matlab function SPath/6dof_system/euler_rate ==
  data: p input; phi_d output; q input; r input; phi input; theta input; theta_d output; psi_d output; psi input
function [phi_d,theta_d,psi_d] = fcn(p,q,r,phi,theta,psi)
    D = [[1 sin(phi)*tan(theta) cos(phi)*tan(theta)];
         [0 cos(phi) -sin(phi)];
         [0 sin(phi)/cos(theta) cos(phi)/cos(theta)]];
    euler_rate = D*[p;q;r]
    phi_d = euler_rate(1)
    theta_d = euler_rate(2)
    psi_d = euler_rate(3)

== matlab function SPath/Controller/ActionDecider/IsRecoverFinish_Detect/MATLAB Function1 ==
  data: u input; y output
function y = fcn(u)
y = 0;
if u == 2
    y = 1;
end

== matlab function SPath/Controller/Sensors/MATLAB Function1 ==
  data: Pos_SensorX1 output; l input; Pos input; Pos_SensorX2 output; Pos_SensorY1 output; m_BtoI input; Pos_SensorY2 output
function [Pos_SensorX1,Pos_SensorX2,Pos_SensorY1,Pos_SensorY2] = fcn(l,Pos,m_BtoI)
    X = Pos(1);
    Y = Pos(2);
    Z = Pos(3);
    
    % Sensor X1 Place
    Sx1_B = [1;0;0]+[0;-1;0];
    Sx1_B = Sx1_B/norm(Sx1_B);
    Sx1_B = l*Sx1_B;
    
    Sx1_I = m_BtoI*Sx1_B;
    Pos_SensorX1 = [X+Sx1_I(1);Y+Sx1_I(2);Z+Sx1_I(3)];
    
    
    % Sensor X2 Place
    Sx2_B = [1;0;0]+[0;1;0];
    Sx2_B = Sx2_B/norm(Sx2_B);
    Sx2_B = l*Sx2_B;
    
    Sx2_I = m_BtoI*Sx2_B;
    Pos_SensorX2 = [X+Sx2_I(1);Y+Sx2_I(2);Z+Sx2_I(3)];
    
    % Sensor Y1 Place
    Sy1_B = [-1;0;0]+[0;-1;0];
    Sy1_B = Sy1_B/norm(Sy1_B);
    Sy1_B = l*Sy1_B;
    
    Sy1_I = m_BtoI*Sy1_B;
    Pos_SensorY1 = [X+Sy1_I(1);Y+Sy1_I(2);Z+Sy1_I(3)];
    
    
    % Sensor Y2 Place
    Sy2_B = [-1;0;0]+[0;1;0];
    Sy2_B = Sy2_B/norm(Sy2_B);
    Sy2_B = l*Sy2_B;
    
    Sy2_I = m_BtoI*Sy2_B;
    Pos_SensorY2 = [X+Sy2_I(1);Y+Sy2_I(2);Z+Sy2_I(3)];

== matlab function SPath/Controller/ActionDecider/IsRecoverFinish_Detect/MATLAB Function2 ==
  data: u input; y output
function y = fcn(u)
y = 0;
if u == 4
    y = 1;
end

== matlab function SPath/Controller/Sensors/SensorY2 ==
  data: Pos input; MinSenseDist output; Bounds input; Yaw input; SenseVect output; MaxRange input
function [MinSenseDist,SenseVect] = fcn(Pos,Bounds,Yaw,MaxRange)
MinSenseDist = MaxRange;
for index = 1:size(Bounds,1)
    Bound = Bounds(index,:);
if length(Pos) > 1
    bx = Bound(1);
    by = Bound(2);
    tx = Bound(3);
    ty = Bound(4);
    X = Pos(1);
    Y = Pos(2);
    Z = Pos(3);
    
    m = [[cos(Yaw) -sin(Yaw)];[sin(Yaw) cos(Yaw)]];
    n = m*[0;1]; % Yb vector
    nx = n(1);
    ny = n(2);

    j = ((ty*bx-tx*by)-(ty*X-tx*Y))/(ty*nx-tx*ny);
    
    if j < 0 % sense backward point
        SenseDist = MaxRange;
    else
        SensePt = [X+nx*j;Y+ny*j];
        
        % Check if ON boundaries
        if tx == 0
            i = (SensePt(2)-by)/ty;
        else
            i = (SensePt(1)-bx)/tx;
        end
        
        % If not
        if i < 0 || i > Bound(7)
            SenseDist = MaxRange;
        % If yes
        else
            SenseDist = sqrt((nx*j)^2 + (ny*j)^2);
        end
    end
    
    SenseVect = [nx;ny;0];
    
else
    SenseDist = MaxRange;
    SenseVect = [0;0;0];
end


if SenseDist < MinSenseDist
    MinSenseDist = SenseDist;
end


end

== matlab function SPath/Controller/Sensors/SensorX1 ==
  data: Pos input; MinSenseDist output; Bounds input; Yaw input; SenseVect output; MaxRange input
function [MinSenseDist,SenseVect] = fcn(Pos,Bounds,Yaw,MaxRange)
MinSenseDist = MaxRange;
for index = 1:size(Bounds,1)
    Bound = Bounds(index,:);
if length(Pos) > 1
    bx = Bound(1);
    by = Bound(2);
    tx = Bound(3);
    ty = Bound(4);
    X = Pos(1);
    Y = Pos(2);
    Z = Pos(3);
    
    m = [[cos(Yaw) -sin(Yaw)];[sin(Yaw) cos(Yaw)]];
    n = m*[1;0]; % Xb vector
    nx = n(1);
    ny = n(2);

    j = ((ty*bx-tx*by)-(ty*X-tx*Y))/(ty*nx-tx*ny);
    
    if j < 0 % sense backward point
        SenseDist = MaxRange;
    else
        SensePt = [X+nx*j;Y+ny*j];
        
        % Check if ON boundaries
        if tx == 0
            i = (SensePt(2)-by)/ty;
        else
            i = (SensePt(1)-bx)/tx;
        end
        
        % If not
        if i < 0 || i > Bound(7)
            SenseDist = MaxRange;
        % If yes
        else
            SenseDist = sqrt((nx*j)^2 + (ny*j)^2);
        end
    end
    
    SenseVect = [nx;ny;0];
    
else
    SenseDist = MaxRange;
    SenseVect = [0;0;0];
end


if SenseDist < MinSenseDist
    MinSenseDist = SenseDist;
end


end

== matlab function SPath/Controller/ActionDecider/IsRecoverFinish_Detect/MATLAB Function ==
  data: mode input; action output; t_md2 input; t_md4 input; ResetFlag output
function [action,ResetFlag] = fcn(mode,t_md2,t_md4)
action = 0;
ResetFlag = 0;
if mode == 4 && t_md4 >= t_md2
    action = -4;
    ResetFlag = 1;
end

== matlab function SPath/Controller/Sensors/SensorX2 ==
  data: Pos input; MinSenseDist output; Bounds input; Yaw input; SenseVect output; MaxRange input
function [MinSenseDist,SenseVect] = fcn(Pos,Bounds,Yaw,MaxRange)
MinSenseDist = MaxRange;
for index = 1:size(Bounds,1)
    Bound = Bounds(index,:);
if length(Pos) > 1
    bx = Bound(1);
    by = Bound(2);
    tx = Bound(3);
    ty = Bound(4);
    X = Pos(1);
    Y = Pos(2);
    Z = Pos(3);
    
    m = [[cos(Yaw) -sin(Yaw)];[sin(Yaw) cos(Yaw)]];
    n = m*[1;0]; % Xb vector
    nx = n(1);
    ny = n(2);

    j = ((ty*bx-tx*by)-(ty*X-tx*Y))/(ty*nx-tx*ny);
    
    if j < 0 % sense backward point
        SenseDist = MaxRange;
    else
        SensePt = [X+nx*j;Y+ny*j];
        
        % Check if ON boundaries
        if tx == 0
            i = (SensePt(2)-by)/ty;
        else
            i = (SensePt(1)-bx)/tx;
        end
        
        % If not
        if i < 0 || i > Bound(7)
            SenseDist = MaxRange;
        % If yes
        else
            SenseDist = sqrt((nx*j)^2 + (ny*j)^2);
        end
    end
    
    SenseVect = [nx;ny;0];
    
else
    SenseDist = MaxRange;
    SenseVect = [0;0;0];
end


if SenseDist < MinSenseDist
    MinSenseDist = SenseDist;
end


end

== matlab function SPath/Force and Environment1/Floor Contact Force/MATLAB Function ==
  data: Thrust input; DetectTakeOff output; m input
function DetectTakeOff = fcn(Thrust,m)
DetectTakeOff = 0;
if Thrust >= m*9.8
    DetectTakeOff = 1;
end

== matlab function SPath/Force and Environment1/Floor Contact Force/MATLAB Function1 ==
  data: IsTakeOff input; N output; Thrust input; m input
function N = fcn(IsTakeOff,Thrust,m)
if IsTakeOff == 0
    N = [0;0;m*9.8-Thrust];
else
    N = [0;0;0];
end

== matlab function SPath/Controller/FlyModeCmd/Normal Fly/TrackYaw ==
  data: Yaw_e input; Yaw_Rate input; mode input; IsYaw input; Detect output
function Detect = fcn(Yaw_e,Yaw_Rate,mode,IsYaw)
% Mode0: Normal Fly
% TrackYawDetect
Detect = 0;
if mode == 0 && IsYaw == 0
    % Should use Flag for the If Yaw Condition.
    if abs(Yaw_e) < 0.05 && abs(Yaw_Rate) < 0.05
        Detect = 1;
    end
end

== matlab function SPath/Controller/Sensors/SensorY1 ==
  data: Pos input; MinSenseDist output; Bounds input; Yaw input; SenseVect output; MaxRange input
function [MinSenseDist,SenseVect] = fcn(Pos,Bounds,Yaw,MaxRange)
MinSenseDist = MaxRange;
for index = 1:size(Bounds,1)
    Bound = Bounds(index,:);
if length(Pos) > 1
    bx = Bound(1);
    by = Bound(2);
    tx = Bound(3);
    ty = Bound(4);
    X = Pos(1);
    Y = Pos(2);
    Z = Pos(3);
    
    m = [[cos(Yaw) -sin(Yaw)];[sin(Yaw) cos(Yaw)]];
    n = m*[0;-1]; % Yb vector
    nx = n(1);
    ny = n(2);

    j = ((ty*bx-tx*by)-(ty*X-tx*Y))/(ty*nx-tx*ny);
    
    if j < 0 % sense backward point
        SenseDist = MaxRange;
    else
        SensePt = [X+nx*j;Y+ny*j];
        
        % Check if ON boundaries
        if tx == 0
            i = (SensePt(2)-by)/ty;
        else
            i = (SensePt(1)-bx)/tx;
        end
        
        % If not
        if i < 0 || i > Bound(7)
            SenseDist = MaxRange;
        % If yes
        else
            SenseDist = sqrt((nx*j)^2 + (ny*j)^2);
        end
    end
    
    SenseVect = [nx;ny;0];
    
else
    SenseDist = MaxRange;
    SenseVect = [0;0;0];
end


if SenseDist < MinSenseDist
    MinSenseDist = SenseDist;
end


end

== matlab function SPath/Controller/ActionDecider/SecondManeuver_Detect/MATLAB Function ==
  data: crosstime input; YVel input; D_SF input; BufferTime output; D_DR input; l input; angle input
function BufferTime = fcn(crosstime,YVel,D_SF,D_DR,l,angle)

if crosstime > 0
    if abs(YVel) >= 0.2
        BufferTime = (D_SF - D_DR - l*cos(angle))/abs(YVel);
    else
        BufferTime = 0.5;
    end
else
    BufferTime = 0.5;
end

== matlab function SPath/Controller/ActionDecider/Recover_Detect/MATLAB Function ==
  data: crosstime input; YVel input; D_SF input; BufferTime output; D_DR input; l input; angle input
function BufferTime = fcn(crosstime,YVel,D_SF,D_DR,l,angle)

if crosstime > 0
    if abs(YVel) >= 0.2
        BufferTime = (D_SF - D_DR - l*cos(angle))/abs(YVel);
    else
        BufferTime = 0.5;
    end
else
    BufferTime = 0.5;
end

== matlab function SPath/Controller/FlyModeCmd/Normal Fly/Variable PD Controller/MATLAB Function ==
  data: u input; P output; D output; N output
function [P,D,N] = fcn(u)
if u > 0.7      % 0.7-[1.0]
    P = 0.45;
    D = 0.75;
    N = 100;
elseif u > 0.3  % 0.3-[0.7]
    P = 0.7;
    D = 0.5;
    N = 20;    
else            % 0.0-0.3
    P = 0.9;
    D = 0.5;
    N = 20;
    
end

== matlab function SPath/Controller/FlyModeCmd/Normal Fly/ForwardFly ==
  data: mode input; IsYaw input; xb_e input; yb_e input; xb_e_cal output; yb_e_cal output
function [xb_e_cal,yb_e_cal]= fcn(mode,IsYaw,xb_e,yb_e)
% Mode0: Normal Fly
xb_e_cal = 0;
yb_e_cal = 0;
if mode == 0
    if IsYaw == 1
        xb_e_cal = 1*xb_e;
        yb_e_cal = 1*yb_e;
    end
end

== matlab function SPath/Controller/FlyModeCmd/MATLAB Function1 ==
  data: WaterLevel input; V_A output
function V_A = fcn(WaterLevel)
x = WaterLevel;

a = -0.0009323;
b = 6.146;
c = 1.17;
d = 0.01205;

V_A = a*exp(b*x) + c*exp(d*x);

== matlab function SPath/Controller/ActionDecider/SecondManeuver_Detect/MATLAB Function1 ==
  data: Hot input; u input; y output
function y = fcn(Hot,u)
if Hot == 1
    y = true;
else
    y = u;
end

== matlab function SPath/Controller/Sensors/MATLAB Function9 ==
  data: S0X output; l input; S0Y output; Vect input
function [S0X,S0Y] = fcn(l,Vect)
MaxRange = 30;
if length(Vect) > 1
    if l == MaxRange
        S0X = MaxRange;
        S0Y = 0;
    else
        nx = Vect(1);
        ny = Vect(2);
        S0X = l*nx;
        S0Y = l*ny;
    end
else 
    S0X = MaxRange;
    S0Y = 0;
end

== matlab function SPath/Controller/ActionDecider/FirstManeuver_Detect/Robust_Design ==
  data: mode input; count output
function count = fcn(mode)
count = 0;
if mode == 1
    count = 1;
end

== matlab function SPath/Controller/ActionDecider/SlowDown_Detect/MATLAB Function7 ==
  data: Accel input; SlowDownDist output; Vx input
function SlowDownDist = fcn(Accel,Vx)
    SlowDownDist = 0.5*Vx^2/Accel;

== matlab function SPath/Controller/ActionDecider/SlowDown_Detect/MATLAB Function11 ==
  data: u input; y output
function y = fcn(u)
    y = 9.8*tan(u);

== matlab function SPath/6dof_system/Drone & Liquid Dynamic Inertia/MATLAB Function ==
  data: hb_ratio input; C_R output
function C_R = fcn(hb_ratio)
x = hb_ratio;
p1 = -1.311;
p2 = 4.077;
p3 = -3.342;
p4 = -0.2563;
p5 = 0.9878;
C_R = p1*x^4 + p2*x^3 + p3*x^2 + p4*x + p5;

== matlab function SPath/Controller/Rotors System1/Motor2Drone ==
  data: FR input; Thrust output; Tq_R output; FL input; BR input; BL input; Tq_P output; Tq_Y output; l input; k input
function [Thrust,Tq_R,Tq_P,Tq_Y] = fcn(FR,FL,BR,BL,l,k)
% Tq_Y needs to change if using the real motor
    l_xy = l/sqrt(2);
    Thrust = FR + FL+ BR + BL;
    Tq_R = (FL+BL)*l_xy - (FR+BR)*l_xy;
    Tq_P = (BL+BR)*l_xy - (FL+FR)*l_xy;
    Tq_Y = (FR+BL)*k - (FL+BR)*k;

== matlab function SPath/6dof_system/ItoBTransform ==
  data: phi input; m output; theta input; psi input
function m = fcn(phi,theta,psi)
    T_ItoV1 = [[cos(psi) sin(psi) 0];[-sin(psi) cos(psi) 0];[0 0 1]]; 
    T_V1toV2 = [[cos(theta) 0 -sin(theta)];[0 1 0];[sin(theta) 0 cos(theta)]];
    T_V2toB = [[1 0 0];[0 cos(phi) sin(phi)];[0 -sin(phi) cos(phi)]];
    m = T_V2toB*T_V1toV2*T_ItoV1

== matlab function SPath/WayPts to XYZerror ==
  data: waypts input; XYZerror output; XYZ input
function XYZerror = fcn(waypts,XYZ)
if length(waypts) > 1
    Xerror = waypts(1)-XYZ(1);
    Yerror = waypts(2)-XYZ(2);
    Zerror = waypts(3)-XYZ(3);
    XYZerror = [Xerror;Yerror;Zerror];
else
    XYZerror = [0;0;0];
end

== matlab function SPath/Controller/Rotors System1/MotorThrustCmd ==
  data: Thrust_Cmd input; FR_Cmd output; FL_Cmd output; BR_Cmd output; BL_Cmd output; Tq_R_Cmd input; Tq_P_Cmd input; Tq_Y_Cmd input; l input; k input
function [FR_Cmd,FL_Cmd,BR_Cmd,BL_Cmd] = fcn(Thrust_Cmd,Tq_R_Cmd,Tq_P_Cmd,Tq_Y_Cmd,l,k)
    N = 4;
    l_xy = l/sqrt(2); % 45 degree configuration
    
    FR_Cmd = Thrust_Cmd/N + Tq_Y_Cmd/(N*k) - Tq_P_Cmd/(N*l_xy) - Tq_R_Cmd/(N*l_xy);
    FL_Cmd = Thrust_Cmd/N - Tq_Y_Cmd/(N*k) - Tq_P_Cmd/(N*l_xy) + Tq_R_Cmd/(N*l_xy);
    BR_Cmd = Thrust_Cmd/N - Tq_Y_Cmd/(N*k) + Tq_P_Cmd/(N*l_xy) - Tq_R_Cmd/(N*l_xy);
    BL_Cmd = Thrust_Cmd/N + Tq_Y_Cmd/(N*k) + Tq_P_Cmd/(N*l_xy) + Tq_R_Cmd/(N*l_xy);
